simulink model "User_Assign_testing"  (R2025a)
settings: Solver=VariableStepAuto  StartTime=0.0  StopTime=10.0  RelTol=1e-3
settings Model: Creator=uss924001  LastModifiedBy=uss924001

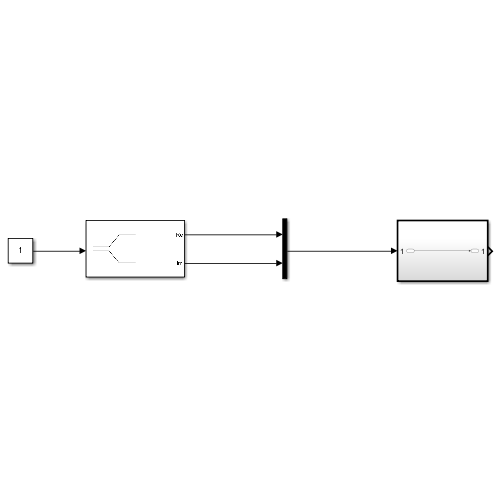
[thumbnail: Simulink's stored preview of the top-level diagram]
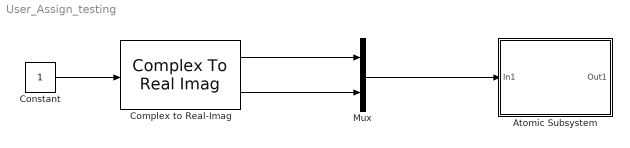
== system User_Assign_testing ==
  Atomic Subsystem : Subsystem  TreatAsAtomicUnit=on
  Complex to Real-Imag : ComplexToRealImag
  Constant : Constant
  Mux : Mux  Inputs=2
  wires:
  Complex to Real-Imag/2 -> Mux/2
  Complex to Real-Imag/1 -> Mux/1
  Constant/1 -> Complex to Real-Imag/1
  Mux/1 -> Atomic Subsystem/1(In1)

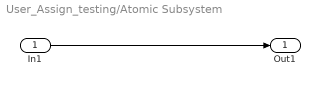
== system User_Assign_testing/Atomic Subsystem ==
  In1 : Inport
  Out1 : Outport
  wires:
  In1/1 -> Out1/1
